simulink model "ground_sim"  (R2022a)
settings: Solver=FixedStepAuto  StartTime=0.0  StopTime=35  FixedStep=framePeriod_s  RelTol=1e-9
values from neighbouring files (symbols this model uses):
  framePeriod_s = 1/frameRate_hz    (= 0.02)    [autocode_setup.m]    (also in setup.m)
undefined symbols (not defined in the file or in its folder): accel_mps2, Aircraft, alt_msl_m, alt_wgs84_m, datetime, datevec, die_temp_c, Earth, Env, Fmu, gyro_radps, hdop, healthy, horz_acc_m, imu_healthy, InitCond, lat_rad, lon_rad, mag_healthy, mag_ut, ned_vel_mps, new_data, new_imu_data, new_mag_data, num_sats, pres_pa, spd_mps, Telem, tow_ms, track_acc_rad, track_rad, vdop, vel_acc_mps, vert_acc_m, week, WGS84
libraries: simulink x8, aerolibconvert2 x5, aerolibasang x3, aerolibtransform2 x2, aerolibgravity2 x2, aerolibatmos2 x1, sharedtransform x1, uavutilslib x1
(part 3 of 4)

== system ground_sim/Flight Management Unit/Vehicle Management System (VMS)/Variant Subsystem/FMU v1/Virtual to Non-Virtual Mapping1/Virtual to Non-Virtual Mapping2 ==
  Virtual : Inport
  Bus Creator : BusCreator  Inputs=new_imu_data,new_mag_data,imu_healthy,mag_healthy,die_temp_c,accel_mps2,gyro_radps,mag_ut  OutDataTypeStr=Bus: ImuData
  Bus Selector : BusSelector  OutputSignals=New IMU Data,New Magnetometer Data,IMU Healthy,Magnetometer Healthy,Die Temperature [C],Accelerometer [m/s/s],Gyro [rad/s],Magnetometer [uT]
  Data Type Conversion{,1..3} (4 alike) : DataTypeConversion  OutDataTypeStr=boolean  SaturateOnIntegerOverflow=off  RndMeth=Floor
  Data Type Conversion{4..7} (4 alike) : DataTypeConversion  OutDataTypeStr=single  SaturateOnIntegerOverflow=off  RndMeth=Floor
  Non-Virtual : Outport  OutDataTypeStr=Bus: ImuData
  wires:
  Bus Creator/1 -> Non-Virtual/1
  Virtual/1 -> Bus Selector/1
  Bus Selector/1 -> Data Type Conversion/1  "<New IMU Data>"
  Data Type Conversion/1 -> Bus Creator/1  "new_imu_data"
  Bus Selector/2 -> Data Type Conversion1/1  "<New Magnetometer Data>"
  Data Type Conversion1/1 -> Bus Creator/2  "new_mag_data"
  Bus Selector/3 -> Data Type Conversion2/1  "<IMU Healthy>"
  Data Type Conversion2/1 -> Bus Creator/3  "imu_healthy"
  Bus Selector/4 -> Data Type Conversion3/1  "<Magnetometer Healthy>"
  Data Type Conversion3/1 -> Bus Creator/4  "mag_healthy"
  Bus Selector/5 -> Data Type Conversion4/1  "<Die Temperature [C]>"
  Data Type Conversion4/1 -> Bus Creator/5  "die_temp_c"
  Bus Selector/6 -> Data Type Conversion5/1  "<Accelerometer [m/s/s]>"
  Bus Selector/7 -> Data Type Conversion6/1  "<Gyro [rad/s]>"
  Bus Selector/8 -> Data Type Conversion7/1  "<Magnetometer [uT]>"
  Data Type Conversion5/1 -> Bus Creator/6  "accel_mps2"
  Data Type Conversion6/1 -> Bus Creator/7  "gyro_radps"
  Data Type Conversion7/1 -> Bus Creator/8  "mag_ut"

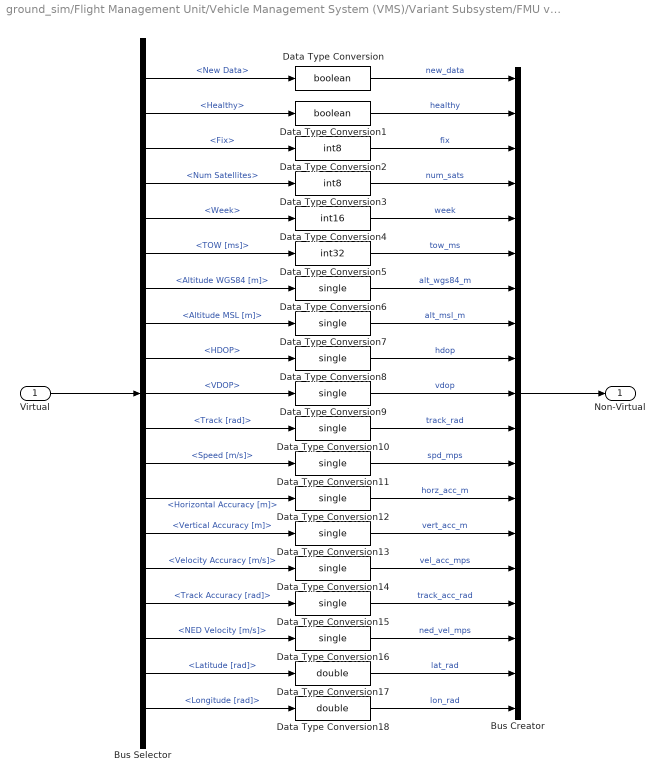
== system ground_sim/Flight Management Unit/Vehicle Management System (VMS)/Variant Subsystem/FMU v1/Virtual to Non-Virtual Mapping1/Virtual to Non-Virtual Mapping3 ==
  Virtual : Inport
  Bus Creator : BusCreator  Inputs=new_data,healthy,fix,num_sats,week,tow_ms,alt_wgs84_m,alt_msl_m,hdop,vdop,track_rad,spd_mps,horz_acc_m,vert_acc_m,vel_acc_mps,track_acc_rad,ned_vel_mps,lat_rad,lon_rad  OutDataTypeStr=Bus: GnssData
  Bus Selector : BusSelector  OutputSignals=New Data,Healthy,Fix,Num Satellites,Week,TOW [ms],Altitude WGS84 [m],Altitude MSL [m],HDOP,VDOP,Track [rad],Speed [m/s],Horizontal Accuracy [m],Vertical Accuracy [m],Velocity Accuracy [m/s],Track Accuracy [rad],NED Velocity [m/s],Latitude [rad],Longitude [rad]
  Data Type Conversion : DataTypeConversion  OutDataTypeStr=boolean  SaturateOnIntegerOverflow=off  RndMeth=Floor
  Data Type Conversion1 : DataTypeConversion  OutDataTypeStr=boolean  SaturateOnIntegerOverflow=off  RndMeth=Floor
  Data Type Conversion{6..16} (11 alike) : DataTypeConversion  OutDataTypeStr=single  SaturateOnIntegerOverflow=off  RndMeth=Floor
  Data Type Conversion17 : DataTypeConversion  OutDataTypeStr=double  SaturateOnIntegerOverflow=off  RndMeth=Floor
  Data Type Conversion18 : DataTypeConversion  OutDataTypeStr=double  SaturateOnIntegerOverflow=off  RndMeth=Floor
  Data Type Conversion2 : DataTypeConversion  OutDataTypeStr=int8  SaturateOnIntegerOverflow=off  RndMeth=Floor
  Data Type Conversion3 : DataTypeConversion  OutDataTypeStr=int8  SaturateOnIntegerOverflow=off  RndMeth=Floor
  Data Type Conversion4 : DataTypeConversion  OutDataTypeStr=int16  SaturateOnIntegerOverflow=off  RndMeth=Floor
  Data Type Conversion5 : DataTypeConversion  OutDataTypeStr=int32  SaturateOnIntegerOverflow=off  RndMeth=Floor
  Non-Virtual : Outport  OutDataTypeStr=Bus: GnssData
  wires:
  Virtual/1 -> Bus Selector/1
  Bus Creator/1 -> Non-Virtual/1
  Bus Selector/1 -> Data Type Conversion/1  "<New Data>"
  Data Type Conversion/1 -> Bus Creator/1  "new_data"
  Bus Selector/2 -> Data Type Conversion1/1  "<Healthy>"
  Data Type Conversion1/1 -> Bus Creator/2  "healthy"
  Bus Selector/3 -> Data Type Conversion2/1  "<Fix>"
  Data Type Conversion2/1 -> Bus Creator/3  "fix"
  Bus Selector/4 -> Data Type Conversion3/1  "<Num Satellites>"
  Data Type Conversion3/1 -> Bus Creator/4  "num_sats"
  Bus Selector/5 -> Data Type Conversion4/1  "<Week>"
  Data Type Conversion4/1 -> Bus Creator/5  "week"
  Bus Selector/6 -> Data Type Conversion5/1  "<TOW [ms]>"
  Data Type Conversion5/1 -> Bus Creator/6  "tow_ms"
  Bus Selector/7 -> Data Type Conversion6/1  "<Altitude WGS84 [m]>"
  Bus Selector/8 -> Data Type Conversion7/1  "<Altitude MSL [m]>"
  Data Type Conversion6/1 -> Bus Creator/7  "alt_wgs84_m"
  Data Type Conversion7/1 -> Bus Creator/8  "alt_msl_m"
  Bus Selector/9 -> Data Type Conversion8/1  "<HDOP>"
  Bus Selector/10 -> Data Type Conversion9/1  "<VDOP>"
  Data Type Conversion8/1 -> Bus Creator/9  "hdop"
  Data Type Conversion9/1 -> Bus Creator/10  "vdop"
  Bus Selector/11 -> Data Type Conversion10/1  "<Track [rad]>"
  Bus Selector/12 -> Data Type Conversion11/1  "<Speed [m/s]>"
  Data Type Conversion10/1 -> Bus Creator/11  "track_rad"
  Data Type Conversion11/1 -> Bus Creator/12  "spd_mps"
  Bus Selector/13 -> Data Type Conversion12/1  "<Horizontal Accuracy [m]>"
  Bus Selector/14 -> Data Type Conversion13/1  "<Vertical Accuracy [m]>"
  Bus Selector/15 -> Data Type Conversion14/1  "<Velocity Accuracy [m/s]>"
  Bus Selector/16 -> Data Type Conversion15/1  "<Track Accuracy [rad]>"
  Bus Selector/17 -> Data Type Conversion16/1  "<NED Velocity [m/s]>"
  Bus Selector/18 -> Data Type Conversion17/1  "<Latitude [rad]>"
  Bus Selector/19 -> Data Type Conversion18/1  "<Longitude [rad]>"
  Data Type Conversion18/1 -> Bus Creator/19  "lon_rad"
  Data Type Conversion17/1 -> Bus Creator/18  "lat_rad"
  Data Type Conversion16/1 -> Bus Creator/17  "ned_vel_mps"
  Data Type Conversion15/1 -> Bus Creator/16  "track_acc_rad"
  Data Type Conversion14/1 -> Bus Creator/15  "vel_acc_mps"
  Data Type Conversion13/1 -> Bus Creator/14  "vert_acc_m"
  Data Type Conversion12/1 -> Bus Creator/13  "horz_acc_m"

== system ground_sim/Flight Management Unit/Vehicle Management System (VMS)/Variant Subsystem/FMU v1/Virtual to Non-Virtual Mapping1/Virtual to Non-Virtual Mapping4 ==
  Virtual : Inport
  Bus Creator : BusCreator  Inputs=new_data,healthy,pres_pa,die_temp_c  OutDataTypeStr=Bus: PresData
  Bus Selector : BusSelector  OutputSignals=New Data,Healthy,Pressure [Pa],Die Temperature [C]
  Data Type Conversion : DataTypeConversion  OutDataTypeStr=boolean  SaturateOnIntegerOverflow=off  RndMeth=Floor
  Data Type Conversion1 : DataTypeConversion  OutDataTypeStr=boolean  SaturateOnIntegerOverflow=off  RndMeth=Floor
  Data Type Conversion2 : DataTypeConversion  OutDataTypeStr=single  SaturateOnIntegerOverflow=off  RndMeth=Floor
  Data Type Conversion3 : DataTypeConversion  OutDataTypeStr=single  SaturateOnIntegerOverflow=off  RndMeth=Floor
  Non-Virtual : Outport  OutDataTypeStr=Bus: PresData
  wires:
  Bus Creator/1 -> Non-Virtual/1
  Virtual/1 -> Bus Selector/1
  Bus Selector/1 -> Data Type Conversion/1  "<New Data>"
  Data Type Conversion/1 -> Bus Creator/1  "new_data"
  Bus Selector/2 -> Data Type Conversion1/1  "<Healthy>"
  Data Type Conversion1/1 -> Bus Creator/2  "healthy"
  Bus Selector/3 -> Data Type Conversion2/1  "<Pressure [Pa]>"
  Data Type Conversion2/1 -> Bus Creator/3  "pres_pa"
  Bus Selector/4 -> Data Type Conversion3/1  "<Die Temperature [C]>"
  Data Type Conversion3/1 -> Bus Creator/4  "die_temp_c"

== system ground_sim/Flight Management Unit/Vehicle Management System (VMS)/Variant Subsystem/FMU v1/Virtual to Non-Virtual Mapping1/Virtual to Non-Virtual Mapping5 ==
  Virtual : Inport
  Bus Creator : BusCreator  Inputs=new_data,healthy,pres_pa,die_temp_c  OutDataTypeStr=Bus: PresData
  Bus Selector : BusSelector  OutputSignals=New Data,Healthy,Pressure [Pa],Die Temperature [C]
  Data Type Conversion : DataTypeConversion  OutDataTypeStr=boolean  SaturateOnIntegerOverflow=off  RndMeth=Floor
  Data Type Conversion1 : DataTypeConversion  OutDataTypeStr=boolean  SaturateOnIntegerOverflow=off  RndMeth=Floor
  Data Type Conversion2 : DataTypeConversion  OutDataTypeStr=single  SaturateOnIntegerOverflow=off  RndMeth=Floor
  Data Type Conversion3 : DataTypeConversion  OutDataTypeStr=single  SaturateOnIntegerOverflow=off  RndMeth=Floor
  Non-Virtual : Outport  OutDataTypeStr=Bus: PresData
  wires:
  Data Type Conversion3/1 -> Bus Creator/4  "die_temp_c"
  Bus Selector/4 -> Data Type Conversion3/1  "<Die Temperature [C]>"
  Data Type Conversion2/1 -> Bus Creator/3  "pres_pa"
  Bus Selector/3 -> Data Type Conversion2/1  "<Pressure [Pa]>"
  Data Type Conversion1/1 -> Bus Creator/2  "healthy"
  Bus Selector/2 -> Data Type Conversion1/1  "<Healthy>"
  Data Type Conversion/1 -> Bus Creator/1  "new_data"
  Bus Selector/1 -> Data Type Conversion/1  "<New Data>"
  Virtual/1 -> Bus Selector/1
  Bus Creator/1 -> Non-Virtual/1

== system ground_sim/Flight Management Unit/Vehicle Management System (VMS)/Variant Subsystem/FMU v1/Virtual to Non-Virtual Mapping1/Virtual to Non-Virtual Mapping6 ==
  Virtual : Inport
  Bus Creator : BusCreator  Inputs=volt  OutDataTypeStr=Bus: AdcData
  Bus Selector : BusSelector  OutputSignals=Voltages
  Data Type Conversion2 : DataTypeConversion  OutDataTypeStr=single  SaturateOnIntegerOverflow=off  RndMeth=Floor
  Non-Virtual : Outport  OutDataTypeStr=Bus: AdcData
  wires:
  Bus Creator/1 -> Non-Virtual/1
  Virtual/1 -> Bus Selector/1
  Data Type Conversion2/1 -> Bus Creator/1  "volt"
  Bus Selector/1 -> Data Type Conversion2/1  "<Voltages>"

== system ground_sim/Flight Management Unit/Vehicle Management System (VMS)/Variant Subsystem/FMU v1/Virtual to Non-Virtual Mapping5/Subsystem2 ==
  Non-Virtual : Inport  OutDataTypeStr=Bus: AnalogData
  Bus Creator : BusCreator  Inputs=1
  Bus Selector : BusSelector  OutputSignals=val
  Data Type Conversion : DataTypeConversion  OutDataTypeStr=double  SaturateOnIntegerOverflow=off  RndMeth=Floor
  Virtual : Outport
  wires:
  Non-Virtual/1 -> Bus Selector/1
  Bus Creator/1 -> Virtual/1
  Data Type Conversion/1 -> Bus Creator/1  "Values"
  Bus Selector/1 -> Data Type Conversion/1  "<val>"

== system ground_sim/Flight Management Unit/Vehicle Management System (VMS)/Variant Subsystem/FMU v1/Virtual to Non-Virtual Mapping5/Subsystem3 ==
  Non-Virtual : Inport  OutDataTypeStr=Bus: PwmCmd
  Bus Creator : BusCreator  Inputs=2
  Bus Selector : BusSelector  OutputSignals=cnt,cmd
  Data Type Conversion : DataTypeConversion  OutDataTypeStr=double  SaturateOnIntegerOverflow=off  RndMeth=Floor
  Data Type Conversion1 : DataTypeConversion  OutDataTypeStr=double  SaturateOnIntegerOverflow=off  RndMeth=Floor
  Virtual : Outport
  wires:
  Non-Virtual/1 -> Bus Selector/1
  Bus Selector/2 -> Data Type Conversion1/1  "<cmd>"
  Data Type Conversion1/1 -> Bus Creator/2  "Cmds"
  Data Type Conversion/1 -> Bus Creator/1  "Counts"
  Bus Selector/1 -> Data Type Conversion/1  "<cnt>"
  Bus Creator/1 -> Virtual/1

== system ground_sim/Flight Management Unit/Vehicle Management System (VMS)/Variant Subsystem/FMU v1/Virtual to Non-Virtual Mapping5/Subsystem4 ==
  Non-Virtual : Inport  OutDataTypeStr=Bus: SbusCmd
  Bus Creator : BusCreator  Inputs=4
  Bus Selector : BusSelector  OutputSignals=ch17,ch18,cnt,cmd
  Data Type Conversion{,1..3} (4 alike) : DataTypeConversion  OutDataTypeStr=double  SaturateOnIntegerOverflow=off  RndMeth=Floor
  Virtual : Outport
  wires:
  Non-Virtual/1 -> Bus Selector/1
  Bus Creator/1 -> Virtual/1
  Bus Selector/1 -> Data Type Conversion/1  "<ch17>"
  Bus Selector/2 -> Data Type Conversion1/1  "<ch18>"
  Bus Selector/3 -> Data Type Conversion2/1  "<cnt>"
  Bus Selector/4 -> Data Type Conversion3/1  "<cmd>"
  Data Type Conversion2/1 -> Bus Creator/3  "Counts"
  Data Type Conversion3/1 -> Bus Creator/4  "Cmds"
  Data Type Conversion1/1 -> Bus Creator/2  "Ch 18"
  Data Type Conversion/1 -> Bus Creator/1  "Ch 17"

== system ground_sim/Flight Management Unit/Vehicle Management System (VMS)/Variant Subsystem/FMU v1/Virtual to Non-Virtual Mapping6/Virtual to Non-Virtual Mapping1 ==
  Virtual : Inport
  Bus Creator : BusCreator  Inputs=6
  Bus Selector : BusSelector  OutputSignals=New Data,Lost Frame,Failsafe,Ch 17,Ch 18,Channel Data
  Data Type Conversion{,1..4} (5 alike) : DataTypeConversion  OutDataTypeStr=boolean  SaturateOnIntegerOverflow=off  RndMeth=Floor
  Data Type Conversion5 : DataTypeConversion  OutDataTypeStr=int16  SaturateOnIntegerOverflow=off  RndMeth=Floor
  Non-Virtual : Outport  OutDataTypeStr=Bus: InceptorData
  wires:
  Virtual/1 -> Bus Selector/1
  Bus Creator/1 -> Non-Virtual/1
  Bus Selector/1 -> Data Type Conversion/1  "<New Data>"
  Bus Selector/2 -> Data Type Conversion1/1  "<Lost Frame>"
  Bus Selector/3 -> Data Type Conversion2/1  "<Failsafe>"
  Bus Selector/4 -> Data Type Conversion3/1  "<Ch 17>"
  Bus Selector/5 -> Data Type Conversion4/1  "<Ch 18>"
  Bus Selector/6 -> Data Type Conversion5/1  "<Channel Data>"
  Data Type Conversion/1 -> Bus Creator/1  "new_data"
  Data Type Conversion1/1 -> Bus Creator/2  "lost_frame"
  Data Type Conversion2/1 -> Bus Creator/3  "failsafe"
  Data Type Conversion3/1 -> Bus Creator/4  "ch17"
  Data Type Conversion4/1 -> Bus Creator/5  "ch18"
  Data Type Conversion5/1 -> Bus Creator/6  "ch"

== system ground_sim/Flight Management Unit/Vehicle Management System (VMS)/Variant Subsystem/FMU v1/Virtual to Non-Virtual Mapping6/Virtual to Non-Virtual Mapping2 ==
  Virtual : Inport
  Bus Creator : BusCreator  Inputs=8
  Bus Selector : BusSelector  OutputSignals=New IMU Data,New Magnetometer Data,IMU Healthy,Magnetometer Healthy,Die Temperature [C],Accelerometer [m/s/s],Gyro [rad/s],Magnetometer [uT]
  Data Type Conversion{,1..3} (4 alike) : DataTypeConversion  OutDataTypeStr=boolean  SaturateOnIntegerOverflow=off  RndMeth=Floor
  Data Type Conversion{4..7} (4 alike) : DataTypeConversion  OutDataTypeStr=single  SaturateOnIntegerOverflow=off  RndMeth=Floor
  Non-Virtual : Outport  OutDataTypeStr=Bus: ImuData
  wires:
  Bus Creator/1 -> Non-Virtual/1
  Virtual/1 -> Bus Selector/1
  Bus Selector/1 -> Data Type Conversion/1  "<New IMU Data>"
  Data Type Conversion/1 -> Bus Creator/1  "new_imu_data"
  Bus Selector/2 -> Data Type Conversion1/1  "<New Magnetometer Data>"
  Data Type Conversion1/1 -> Bus Creator/2  "new_mag_data"
  Bus Selector/3 -> Data Type Conversion2/1  "<IMU Healthy>"
  Data Type Conversion2/1 -> Bus Creator/3  "imu_healthy"
  Bus Selector/4 -> Data Type Conversion3/1  "<Magnetometer Healthy>"
  Data Type Conversion3/1 -> Bus Creator/4  "mag_healthy"
  Bus Selector/5 -> Data Type Conversion4/1  "<Die Temperature [C]>"
  Data Type Conversion4/1 -> Bus Creator/5  "die_temp_c"
  Bus Selector/6 -> Data Type Conversion5/1  "<Accelerometer [m/s/s]>"
  Bus Selector/7 -> Data Type Conversion6/1  "<Gyro [rad/s]>"
  Bus Selector/8 -> Data Type Conversion7/1  "<Magnetometer [uT]>"
  Data Type Conversion5/1 -> Bus Creator/6  "accel_mps2"
  Data Type Conversion6/1 -> Bus Creator/7  "gyro_radps"
  Data Type Conversion7/1 -> Bus Creator/8  "mag_ut"

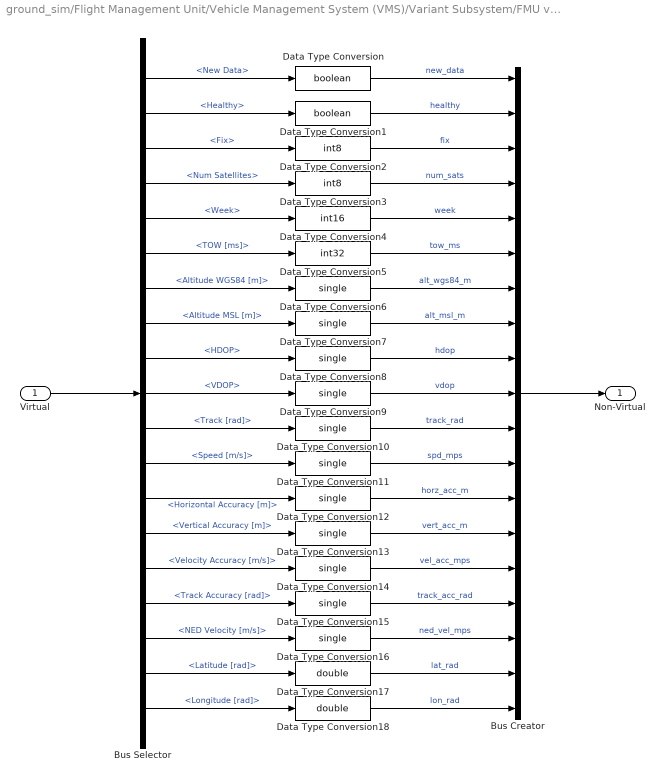
== system ground_sim/Flight Management Unit/Vehicle Management System (VMS)/Variant Subsystem/FMU v1/Virtual to Non-Virtual Mapping6/Virtual to Non-Virtual Mapping3 ==
  Virtual : Inport
  Bus Creator : BusCreator  Inputs=19
  Bus Selector : BusSelector  OutputSignals=New Data,Healthy,Fix,Num Satellites,Week,TOW [ms],Altitude WGS84 [m],Altitude MSL [m],HDOP,VDOP,Track [rad],Speed [m/s],Horizontal Accuracy [m],Vertical Accuracy [m],Velocity Accuracy [m/s],Track Accuracy [rad],NED Velocity [m/s],Latitude [rad],Longitude [rad]
  Data Type Conversion : DataTypeConversion  OutDataTypeStr=boolean  SaturateOnIntegerOverflow=off  RndMeth=Floor
  Data Type Conversion1 : DataTypeConversion  OutDataTypeStr=boolean  SaturateOnIntegerOverflow=off  RndMeth=Floor
  Data Type Conversion{6..16} (11 alike) : DataTypeConversion  OutDataTypeStr=single  SaturateOnIntegerOverflow=off  RndMeth=Floor
  Data Type Conversion17 : DataTypeConversion  OutDataTypeStr=double  SaturateOnIntegerOverflow=off  RndMeth=Floor
  Data Type Conversion18 : DataTypeConversion  OutDataTypeStr=double  SaturateOnIntegerOverflow=off  RndMeth=Floor
  Data Type Conversion2 : DataTypeConversion  OutDataTypeStr=int8  SaturateOnIntegerOverflow=off  RndMeth=Floor
  Data Type Conversion3 : DataTypeConversion  OutDataTypeStr=int8  SaturateOnIntegerOverflow=off  RndMeth=Floor
  Data Type Conversion4 : DataTypeConversion  OutDataTypeStr=int16  SaturateOnIntegerOverflow=off  RndMeth=Floor
  Data Type Conversion5 : DataTypeConversion  OutDataTypeStr=int32  SaturateOnIntegerOverflow=off  RndMeth=Floor
  Non-Virtual : Outport  OutDataTypeStr=Bus: GnssData
  wires:
  Virtual/1 -> Bus Selector/1
  Bus Creator/1 -> Non-Virtual/1
  Bus Selector/1 -> Data Type Conversion/1  "<New Data>"
  Data Type Conversion/1 -> Bus Creator/1  "new_data"
  Bus Selector/2 -> Data Type Conversion1/1  "<Healthy>"
  Data Type Conversion1/1 -> Bus Creator/2  "healthy"
  Bus Selector/3 -> Data Type Conversion2/1  "<Fix>"
  Data Type Conversion2/1 -> Bus Creator/3  "fix"
  Bus Selector/4 -> Data Type Conversion3/1  "<Num Satellites>"
  Data Type Conversion3/1 -> Bus Creator/4  "num_sats"
  Bus Selector/5 -> Data Type Conversion4/1  "<Week>"
  Data Type Conversion4/1 -> Bus Creator/5  "week"
  Bus Selector/6 -> Data Type Conversion5/1  "<TOW [ms]>"
  Data Type Conversion5/1 -> Bus Creator/6  "tow_ms"
  Bus Selector/7 -> Data Type Conversion6/1  "<Altitude WGS84 [m]>"
  Bus Selector/8 -> Data Type Conversion7/1  "<Altitude MSL [m]>"
  Data Type Conversion6/1 -> Bus Creator/7  "alt_wgs84_m"
  Data Type Conversion7/1 -> Bus Creator/8  "alt_msl_m"
  Bus Selector/9 -> Data Type Conversion8/1  "<HDOP>"
  Bus Selector/10 -> Data Type Conversion9/1  "<VDOP>"
  Data Type Conversion8/1 -> Bus Creator/9  "hdop"
  Data Type Conversion9/1 -> Bus Creator/10  "vdop"
  Bus Selector/11 -> Data Type Conversion10/1  "<Track [rad]>"
  Bus Selector/12 -> Data Type Conversion11/1  "<Speed [m/s]>"
  Data Type Conversion10/1 -> Bus Creator/11  "track_rad"
  Data Type Conversion11/1 -> Bus Creator/12  "spd_mps"
  Bus Selector/13 -> Data Type Conversion12/1  "<Horizontal Accuracy [m]>"
  Bus Selector/14 -> Data Type Conversion13/1  "<Vertical Accuracy [m]>"
  Bus Selector/15 -> Data Type Conversion14/1  "<Velocity Accuracy [m/s]>"
  Bus Selector/16 -> Data Type Conversion15/1  "<Track Accuracy [rad]>"
  Bus Selector/17 -> Data Type Conversion16/1  "<NED Velocity [m/s]>"
  Bus Selector/18 -> Data Type Conversion17/1  "<Latitude [rad]>"
  Bus Selector/19 -> Data Type Conversion18/1  "<Longitude [rad]>"
  Data Type Conversion18/1 -> Bus Creator/19  "lon_rad"
  Data Type Conversion17/1 -> Bus Creator/18  "lat_rad"
  Data Type Conversion16/1 -> Bus Creator/17  "ned_vel_mps"
  Data Type Conversion15/1 -> Bus Creator/16  "track_acc_rad"
  Data Type Conversion14/1 -> Bus Creator/15  "vel_acc_mps"
  Data Type Conversion13/1 -> Bus Creator/14  "vert_acc_m"
  Data Type Conversion12/1 -> Bus Creator/13  "horz_acc_m"

== system ground_sim/Flight Management Unit/Vehicle Management System (VMS)/Variant Subsystem/FMU v1/Virtual to Non-Virtual Mapping6/Virtual to Non-Virtual Mapping4 ==
  Virtual : Inport
  Bus Creator : BusCreator  Inputs=4
  Bus Selector : BusSelector  OutputSignals=New Data,Healthy,Pressure [Pa],Die Temperature [C]
  Data Type Conversion : DataTypeConversion  OutDataTypeStr=boolean  SaturateOnIntegerOverflow=off  RndMeth=Floor
  Data Type Conversion1 : DataTypeConversion  OutDataTypeStr=boolean  SaturateOnIntegerOverflow=off  RndMeth=Floor
  Data Type Conversion2 : DataTypeConversion  OutDataTypeStr=single  SaturateOnIntegerOverflow=off  RndMeth=Floor
  Data Type Conversion3 : DataTypeConversion  OutDataTypeStr=single  SaturateOnIntegerOverflow=off  RndMeth=Floor
  Non-Virtual : Outport  OutDataTypeStr=Bus: PresData
  wires:
  Bus Creator/1 -> Non-Virtual/1
  Virtual/1 -> Bus Selector/1
  Bus Selector/1 -> Data Type Conversion/1  "<New Data>"
  Data Type Conversion/1 -> Bus Creator/1  "new_data"
  Bus Selector/2 -> Data Type Conversion1/1  "<Healthy>"
  Data Type Conversion1/1 -> Bus Creator/2  "healthy"
  Bus Selector/3 -> Data Type Conversion2/1  "<Pressure [Pa]>"
  Data Type Conversion2/1 -> Bus Creator/3  "pres_pa"
  Bus Selector/4 -> Data Type Conversion3/1  "<Die Temperature [C]>"
  Data Type Conversion3/1 -> Bus Creator/4  "die_temp_c"

== system ground_sim/Flight Management Unit/Vehicle Management System (VMS)/Variant Subsystem/FMU v1/Virtual to Non-Virtual Mapping6/Virtual to Non-Virtual Mapping5 ==
  Virtual : Inport
  Bus Creator : BusCreator  Inputs=4
  Bus Selector : BusSelector  OutputSignals=New Data,Healthy,Pressure [Pa],Die Temperature [C]
  Data Type Conversion : DataTypeConversion  OutDataTypeStr=boolean  SaturateOnIntegerOverflow=off  RndMeth=Floor
  Data Type Conversion1 : DataTypeConversion  OutDataTypeStr=boolean  SaturateOnIntegerOverflow=off  RndMeth=Floor
  Data Type Conversion2 : DataTypeConversion  OutDataTypeStr=single  SaturateOnIntegerOverflow=off  RndMeth=Floor
  Data Type Conversion3 : DataTypeConversion  OutDataTypeStr=single  SaturateOnIntegerOverflow=off  RndMeth=Floor
  Non-Virtual : Outport  OutDataTypeStr=Bus: PresData
  wires:
  Data Type Conversion3/1 -> Bus Creator/4  "die_temp_c"
  Bus Selector/4 -> Data Type Conversion3/1  "<Die Temperature [C]>"
  Data Type Conversion2/1 -> Bus Creator/3  "pres_pa"
  Bus Selector/3 -> Data Type Conversion2/1  "<Pressure [Pa]>"
  Data Type Conversion1/1 -> Bus Creator/2  "healthy"
  Bus Selector/2 -> Data Type Conversion1/1  "<Healthy>"
  Data Type Conversion/1 -> Bus Creator/1  "new_data"
  Bus Selector/1 -> Data Type Conversion/1  "<New Data>"
  Virtual/1 -> Bus Selector/1
  Bus Creator/1 -> Non-Virtual/1

== system ground_sim/Flight Management Unit/Vehicle Management System (VMS)/Variant Subsystem/FMU v1/Virtual to Non-Virtual Mapping6/Virtual to Non-Virtual Mapping6 ==
  Virtual : Inport
  Bus Creator : BusCreator  Inputs=1
  Bus Selector : BusSelector  OutputSignals=Voltages
  Data Type Conversion2 : DataTypeConversion  OutDataTypeStr=single  SaturateOnIntegerOverflow=off  RndMeth=Floor
  Non-Virtual : Outport  OutDataTypeStr=Bus: AdcData
  wires:
  Bus Creator/1 -> Non-Virtual/1
  Virtual/1 -> Bus Selector/1
  Data Type Conversion2/1 -> Bus Creator/1  "volt"
  Bus Selector/1 -> Data Type Conversion2/1  "<Voltages>"

== system ground_sim/Flight Management Unit/Vehicle Management System (VMS)/Variant Subsystem/FMU v1/Virtual to Non-Virtual Mapping6/Virtual to Non-Virtual Mapping7 ==
  Virtual : Inport
  Bus Creator : BusCreator  Inputs=2
  Bus Selector : BusSelector  OutputSignals=Voltage [V],Current [V]
  Data Type Conversion1 : DataTypeConversion  OutDataTypeStr=single  SaturateOnIntegerOverflow=off  RndMeth=Floor
  Data Type Conversion2 : DataTypeConversion  OutDataTypeStr=single  SaturateOnIntegerOverflow=off  RndMeth=Floor
  Non-Virtual : Outport  OutDataTypeStr=Bus: PowerModuleData
  wires:
  Virtual/1 -> Bus Selector/1
  Bus Creator/1 -> Non-Virtual/1
  Bus Selector/1 -> Data Type Conversion1/1  "<Voltage [V]>"
  Data Type Conversion1/1 -> Bus Creator/1  "voltage_v"
  Bus Selector/2 -> Data Type Conversion2/1  "<Current [V]>"
  Data Type Conversion2/1 -> Bus Creator/2  "current_v"

== system ground_sim/Flight Management Unit/Vehicle Management System (VMS)/Variant Subsystem/FMU v2/Virtual to Non-Virtual Mapping1/Virtual to Non-Virtual Mapping1 ==
  Virtual : Inport
  Bus Creator : BusCreator  Inputs=6
  Bus Selector : BusSelector  OutputSignals=New Data,Lost Frame,Failsafe,Ch 17,Ch 18,Channel Data
  Data Type Conversion{,1..4} (5 alike) : DataTypeConversion  OutDataTypeStr=boolean  SaturateOnIntegerOverflow=off  RndMeth=Floor
  Data Type Conversion5 : DataTypeConversion  OutDataTypeStr=int16  SaturateOnIntegerOverflow=off  RndMeth=Floor
  Non-Virtual : Outport  OutDataTypeStr=Bus: InceptorData
  wires:
  Virtual/1 -> Bus Selector/1
  Bus Creator/1 -> Non-Virtual/1
  Bus Selector/1 -> Data Type Conversion/1  "<New Data>"
  Bus Selector/2 -> Data Type Conversion1/1  "<Lost Frame>"
  Bus Selector/3 -> Data Type Conversion2/1  "<Failsafe>"
  Bus Selector/4 -> Data Type Conversion3/1  "<Ch 17>"
  Bus Selector/5 -> Data Type Conversion4/1  "<Ch 18>"
  Bus Selector/6 -> Data Type Conversion5/1  "<Channel Data>"
  Data Type Conversion/1 -> Bus Creator/1  "new_data"
  Data Type Conversion1/1 -> Bus Creator/2  "lost_frame"
  Data Type Conversion2/1 -> Bus Creator/3  "failsafe"
  Data Type Conversion3/1 -> Bus Creator/4  "ch17"
  Data Type Conversion4/1 -> Bus Creator/5  "ch18"
  Data Type Conversion5/1 -> Bus Creator/6  "ch"

== system ground_sim/Flight Management Unit/Vehicle Management System (VMS)/Variant Subsystem/FMU v2/Virtual to Non-Virtual Mapping1/Virtual to Non-Virtual Mapping2 ==
  Virtual : Inport
  Bus Creator : BusCreator  Inputs=8
  Bus Selector : BusSelector  OutputSignals=New IMU Data,New Magnetometer Data,IMU Healthy,Magnetometer Healthy,Die Temperature [C],Accelerometer [m/s/s],Gyro [rad/s],Magnetometer [uT]
  Data Type Conversion{,1..3} (4 alike) : DataTypeConversion  OutDataTypeStr=boolean  SaturateOnIntegerOverflow=off  RndMeth=Floor
  Data Type Conversion{4..7} (4 alike) : DataTypeConversion  OutDataTypeStr=single  SaturateOnIntegerOverflow=off  RndMeth=Floor
  Non-Virtual : Outport  OutDataTypeStr=Bus: ImuData
  wires:
  Bus Creator/1 -> Non-Virtual/1
  Virtual/1 -> Bus Selector/1
  Bus Selector/1 -> Data Type Conversion/1  "<New IMU Data>"
  Data Type Conversion/1 -> Bus Creator/1  "new_imu_data"
  Bus Selector/2 -> Data Type Conversion1/1  "<New Magnetometer Data>"
  Data Type Conversion1/1 -> Bus Creator/2  "new_mag_data"
  Bus Selector/3 -> Data Type Conversion2/1  "<IMU Healthy>"
  Data Type Conversion2/1 -> Bus Creator/3  "imu_healthy"
  Bus Selector/4 -> Data Type Conversion3/1  "<Magnetometer Healthy>"
  Data Type Conversion3/1 -> Bus Creator/4  "mag_healthy"
  Bus Selector/5 -> Data Type Conversion4/1  "<Die Temperature [C]>"
  Data Type Conversion4/1 -> Bus Creator/5  "die_temp_c"
  Bus Selector/6 -> Data Type Conversion5/1  "<Accelerometer [m/s/s]>"
  Bus Selector/7 -> Data Type Conversion6/1  "<Gyro [rad/s]>"
  Bus Selector/8 -> Data Type Conversion7/1  "<Magnetometer [uT]>"
  Data Type Conversion5/1 -> Bus Creator/6  "accel_mps2"
  Data Type Conversion6/1 -> Bus Creator/7  "gyro_radps"
  Data Type Conversion7/1 -> Bus Creator/8  "mag_ut"

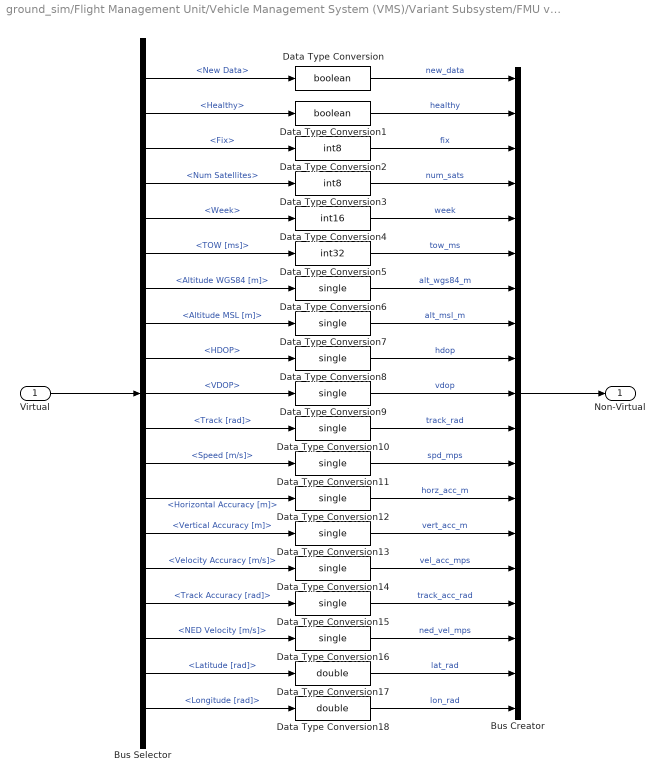
== system ground_sim/Flight Management Unit/Vehicle Management System (VMS)/Variant Subsystem/FMU v2/Virtual to Non-Virtual Mapping1/Virtual to Non-Virtual Mapping3 ==
  Virtual : Inport
  Bus Creator : BusCreator  Inputs=19
  Bus Selector : BusSelector  OutputSignals=New Data,Healthy,Fix,Num Satellites,Week,TOW [ms],Altitude WGS84 [m],Altitude MSL [m],HDOP,VDOP,Track [rad],Speed [m/s],Horizontal Accuracy [m],Vertical Accuracy [m],Velocity Accuracy [m/s],Track Accuracy [rad],NED Velocity [m/s],Latitude [rad],Longitude [rad]
  Data Type Conversion : DataTypeConversion  OutDataTypeStr=boolean  SaturateOnIntegerOverflow=off  RndMeth=Floor
  Data Type Conversion1 : DataTypeConversion  OutDataTypeStr=boolean  SaturateOnIntegerOverflow=off  RndMeth=Floor
  Data Type Conversion{6..16} (11 alike) : DataTypeConversion  OutDataTypeStr=single  SaturateOnIntegerOverflow=off  RndMeth=Floor
  Data Type Conversion17 : DataTypeConversion  OutDataTypeStr=double  SaturateOnIntegerOverflow=off  RndMeth=Floor
  Data Type Conversion18 : DataTypeConversion  OutDataTypeStr=double  SaturateOnIntegerOverflow=off  RndMeth=Floor
  Data Type Conversion2 : DataTypeConversion  OutDataTypeStr=int8  SaturateOnIntegerOverflow=off  RndMeth=Floor
  Data Type Conversion3 : DataTypeConversion  OutDataTypeStr=int8  SaturateOnIntegerOverflow=off  RndMeth=Floor
  Data Type Conversion4 : DataTypeConversion  OutDataTypeStr=int16  SaturateOnIntegerOverflow=off  RndMeth=Floor
  Data Type Conversion5 : DataTypeConversion  OutDataTypeStr=int32  SaturateOnIntegerOverflow=off  RndMeth=Floor
  Non-Virtual : Outport  OutDataTypeStr=Bus: GnssData
  wires:
  Virtual/1 -> Bus Selector/1
  Bus Creator/1 -> Non-Virtual/1
  Bus Selector/1 -> Data Type Conversion/1  "<New Data>"
  Data Type Conversion/1 -> Bus Creator/1  "new_data"
  Bus Selector/2 -> Data Type Conversion1/1  "<Healthy>"
  Data Type Conversion1/1 -> Bus Creator/2  "healthy"
  Bus Selector/3 -> Data Type Conversion2/1  "<Fix>"
  Data Type Conversion2/1 -> Bus Creator/3  "fix"
  Bus Selector/4 -> Data Type Conversion3/1  "<Num Satellites>"
  Data Type Conversion3/1 -> Bus Creator/4  "num_sats"
  Bus Selector/5 -> Data Type Conversion4/1  "<Week>"
  Data Type Conversion4/1 -> Bus Creator/5  "week"
  Bus Selector/6 -> Data Type Conversion5/1  "<TOW [ms]>"
  Data Type Conversion5/1 -> Bus Creator/6  "tow_ms"
  Bus Selector/7 -> Data Type Conversion6/1  "<Altitude WGS84 [m]>"
  Bus Selector/8 -> Data Type Conversion7/1  "<Altitude MSL [m]>"
  Data Type Conversion6/1 -> Bus Creator/7  "alt_wgs84_m"
  Data Type Conversion7/1 -> Bus Creator/8  "alt_msl_m"
  Bus Selector/9 -> Data Type Conversion8/1  "<HDOP>"
  Bus Selector/10 -> Data Type Conversion9/1  "<VDOP>"
  Data Type Conversion8/1 -> Bus Creator/9  "hdop"
  Data Type Conversion9/1 -> Bus Creator/10  "vdop"
  Bus Selector/11 -> Data Type Conversion10/1  "<Track [rad]>"
  Bus Selector/12 -> Data Type Conversion11/1  "<Speed [m/s]>"
  Data Type Conversion10/1 -> Bus Creator/11  "track_rad"
  Data Type Conversion11/1 -> Bus Creator/12  "spd_mps"
  Bus Selector/13 -> Data Type Conversion12/1  "<Horizontal Accuracy [m]>"
  Bus Selector/14 -> Data Type Conversion13/1  "<Vertical Accuracy [m]>"
  Bus Selector/15 -> Data Type Conversion14/1  "<Velocity Accuracy [m/s]>"
  Bus Selector/16 -> Data Type Conversion15/1  "<Track Accuracy [rad]>"
  Bus Selector/17 -> Data Type Conversion16/1  "<NED Velocity [m/s]>"
  Bus Selector/18 -> Data Type Conversion17/1  "<Latitude [rad]>"
  Bus Selector/19 -> Data Type Conversion18/1  "<Longitude [rad]>"
  Data Type Conversion18/1 -> Bus Creator/19  "lon_rad"
  Data Type Conversion17/1 -> Bus Creator/18  "lat_rad"
  Data Type Conversion16/1 -> Bus Creator/17  "ned_vel_mps"
  Data Type Conversion15/1 -> Bus Creator/16  "track_acc_rad"
  Data Type Conversion14/1 -> Bus Creator/15  "vel_acc_mps"
  Data Type Conversion13/1 -> Bus Creator/14  "vert_acc_m"
  Data Type Conversion12/1 -> Bus Creator/13  "horz_acc_m"

== system ground_sim/Flight Management Unit/Vehicle Management System (VMS)/Variant Subsystem/FMU v2/Virtual to Non-Virtual Mapping1/Virtual to Non-Virtual Mapping4 ==
  Virtual : Inport
  Bus Creator : BusCreator  Inputs=4
  Bus Selector : BusSelector  OutputSignals=New Data,Healthy,Pressure [Pa],Die Temperature [C]
  Data Type Conversion : DataTypeConversion  OutDataTypeStr=boolean  SaturateOnIntegerOverflow=off  RndMeth=Floor
  Data Type Conversion1 : DataTypeConversion  OutDataTypeStr=boolean  SaturateOnIntegerOverflow=off  RndMeth=Floor
  Data Type Conversion2 : DataTypeConversion  OutDataTypeStr=single  SaturateOnIntegerOverflow=off  RndMeth=Floor
  Data Type Conversion3 : DataTypeConversion  OutDataTypeStr=single  SaturateOnIntegerOverflow=off  RndMeth=Floor
  Non-Virtual : Outport  OutDataTypeStr=Bus: PresData
  wires:
  Bus Creator/1 -> Non-Virtual/1
  Virtual/1 -> Bus Selector/1
  Bus Selector/1 -> Data Type Conversion/1  "<New Data>"
  Data Type Conversion/1 -> Bus Creator/1  "new_data"
  Bus Selector/2 -> Data Type Conversion1/1  "<Healthy>"
  Data Type Conversion1/1 -> Bus Creator/2  "healthy"
  Bus Selector/3 -> Data Type Conversion2/1  "<Pressure [Pa]>"
  Data Type Conversion2/1 -> Bus Creator/3  "pres_pa"
  Bus Selector/4 -> Data Type Conversion3/1  "<Die Temperature [C]>"
  Data Type Conversion3/1 -> Bus Creator/4  "die_temp_c"

== system ground_sim/Flight Management Unit/Vehicle Management System (VMS)/Variant Subsystem/FMU v2/Virtual to Non-Virtual Mapping1/Virtual to Non-Virtual Mapping5 ==
  Virtual : Inport
  Bus Creator : BusCreator  Inputs=4
  Bus Selector : BusSelector  OutputSignals=New Data,Healthy,Pressure [Pa],Die Temperature [C]
  Data Type Conversion : DataTypeConversion  OutDataTypeStr=boolean  SaturateOnIntegerOverflow=off  RndMeth=Floor
  Data Type Conversion1 : DataTypeConversion  OutDataTypeStr=boolean  SaturateOnIntegerOverflow=off  RndMeth=Floor
  Data Type Conversion2 : DataTypeConversion  OutDataTypeStr=single  SaturateOnIntegerOverflow=off  RndMeth=Floor
  Data Type Conversion3 : DataTypeConversion  OutDataTypeStr=single  SaturateOnIntegerOverflow=off  RndMeth=Floor
  Non-Virtual : Outport  OutDataTypeStr=Bus: PresData
  wires:
  Data Type Conversion3/1 -> Bus Creator/4  "die_temp_c"
  Bus Selector/4 -> Data Type Conversion3/1  "<Die Temperature [C]>"
  Data Type Conversion2/1 -> Bus Creator/3  "pres_pa"
  Bus Selector/3 -> Data Type Conversion2/1  "<Pressure [Pa]>"
  Data Type Conversion1/1 -> Bus Creator/2  "healthy"
  Bus Selector/2 -> Data Type Conversion1/1  "<Healthy>"
  Data Type Conversion/1 -> Bus Creator/1  "new_data"
  Bus Selector/1 -> Data Type Conversion/1  "<New Data>"
  Virtual/1 -> Bus Selector/1
  Bus Creator/1 -> Non-Virtual/1

== system ground_sim/Flight Management Unit/Vehicle Management System (VMS)/Variant Subsystem/FMU v2/Virtual to Non-Virtual Mapping1/Virtual to Non-Virtual Mapping6 ==
  Virtual : Inport
  Bus Creator : BusCreator  Inputs=1
  Bus Selector : BusSelector  OutputSignals=Voltages
  Data Type Conversion2 : DataTypeConversion  OutDataTypeStr=single  SaturateOnIntegerOverflow=off  RndMeth=Floor
  Non-Virtual : Outport  OutDataTypeStr=Bus: AdcData
  wires:
  Bus Creator/1 -> Non-Virtual/1
  Virtual/1 -> Bus Selector/1
  Data Type Conversion2/1 -> Bus Creator/1  "volt"
  Bus Selector/1 -> Data Type Conversion2/1  "<Voltages>"

== system ground_sim/Flight Management Unit/Vehicle Management System (VMS)/Variant Subsystem/FMU v2/Virtual to Non-Virtual Mapping1/Virtual to Non-Virtual Mapping7 ==
  Virtual : Inport
  Bus Creator : BusCreator  Inputs=2
  Bus Selector : BusSelector  OutputSignals=Voltage [V],Current [V]
  Data Type Conversion1 : DataTypeConversion  OutDataTypeStr=single  SaturateOnIntegerOverflow=off  RndMeth=Floor
  Data Type Conversion2 : DataTypeConversion  OutDataTypeStr=single  SaturateOnIntegerOverflow=off  RndMeth=Floor
  Non-Virtual : Outport  OutDataTypeStr=Bus: PowerModuleData
  wires:
  Virtual/1 -> Bus Selector/1
  Bus Creator/1 -> Non-Virtual/1
  Bus Selector/1 -> Data Type Conversion1/1  "<Voltage [V]>"
  Data Type Conversion1/1 -> Bus Creator/1  "voltage_v"
  Bus Selector/2 -> Data Type Conversion2/1  "<Current [V]>"
  Data Type Conversion2/1 -> Bus Creator/2  "current_v"

== system ground_sim/Flight Management Unit/Vehicle Management System (VMS)/Variant Subsystem/FMU v2/Virtual to Non-Virtual Mapping4/Subsystem1 ==
  Non-Virtual : Inport  OutDataTypeStr=Bus: BatteryData
  Bus Creator : BusCreator  Inputs=5
  Bus Selector : BusSelector  OutputSignals=voltage_v,current_ma,consumed_mah,remaining_prcnt,remaining_time_s
  Data Type Conversion{,1..4} (5 alike) : DataTypeConversion  OutDataTypeStr=double  SaturateOnIntegerOverflow=off  RndMeth=Floor
  Virtual : Outport
  wires:
  Non-Virtual/1 -> Bus Selector/1
  Bus Selector/1 -> Data Type Conversion/1  "<voltage_v>"
  Bus Selector/2 -> Data Type Conversion1/1  "<current_ma>"
  Bus Selector/3 -> Data Type Conversion2/1  "<consumed_mah>"
  Bus Selector/4 -> Data Type Conversion3/1  "<remaining_prcnt>"
  Bus Selector/5 -> Data Type Conversion4/1  "<remaining_time_s>"
  Bus Creator/1 -> Virtual/1
  Data Type Conversion/1 -> Bus Creator/1  "Voltage [V]"
  Data Type Conversion1/1 -> Bus Creator/2  "Current [mA]"
  Data Type Conversion2/1 -> Bus Creator/3  "Consumed Capacity [mAh]"
  Data Type Conversion3/1 -> Bus Creator/4  "Remaining Capacity [%]"
  Data Type Conversion4/1 -> Bus Creator/5  "Remaining Flight Time [s]"

== system ground_sim/Flight Management Unit/Vehicle Management System (VMS)/Variant Subsystem/FMU v2/Virtual to Non-Virtual Mapping4/Subsystem2 ==
  Non-Virtual : Inport  OutDataTypeStr=Bus: AnalogData
  Bus Creator : BusCreator  Inputs=1
  Bus Selector : BusSelector  OutputSignals=val
  Data Type Conversion : DataTypeConversion  OutDataTypeStr=double  SaturateOnIntegerOverflow=off  RndMeth=Floor
  Virtual : Outport
  wires:
  Non-Virtual/1 -> Bus Selector/1
  Bus Creator/1 -> Virtual/1
  Data Type Conversion/1 -> Bus Creator/1  "Values"
  Bus Selector/1 -> Data Type Conversion/1  "<val>"

== system ground_sim/Flight Management Unit/Vehicle Management System (VMS)/Variant Subsystem/FMU v2/Virtual to Non-Virtual Mapping4/Subsystem3 ==
  Non-Virtual : Inport  OutDataTypeStr=Bus: PwmCmd
  Bus Creator : BusCreator  Inputs=2
  Bus Selector : BusSelector  OutputSignals=cnt,cmd
  Data Type Conversion : DataTypeConversion  OutDataTypeStr=double  SaturateOnIntegerOverflow=off  RndMeth=Floor
  Data Type Conversion1 : DataTypeConversion  OutDataTypeStr=double  SaturateOnIntegerOverflow=off  RndMeth=Floor
  Virtual : Outport
  wires:
  Non-Virtual/1 -> Bus Selector/1
  Bus Selector/2 -> Data Type Conversion1/1  "<cmd>"
  Data Type Conversion1/1 -> Bus Creator/2  "Cmds"
  Data Type Conversion/1 -> Bus Creator/1  "Counts"
  Bus Selector/1 -> Data Type Conversion/1  "<cnt>"
  Bus Creator/1 -> Virtual/1

== system ground_sim/Flight Management Unit/Vehicle Management System (VMS)/Variant Subsystem/FMU v2/Virtual to Non-Virtual Mapping4/Subsystem4 ==
  Non-Virtual : Inport  OutDataTypeStr=Bus: SbusCmd
  Bus Creator : BusCreator  Inputs=4
  Bus Selector : BusSelector  OutputSignals=ch17,ch18,cnt,cmd
  Data Type Conversion{,1..3} (4 alike) : DataTypeConversion  OutDataTypeStr=double  SaturateOnIntegerOverflow=off  RndMeth=Floor
  Virtual : Outport
  wires:
  Non-Virtual/1 -> Bus Selector/1
  Bus Creator/1 -> Virtual/1
  Bus Selector/1 -> Data Type Conversion/1  "<ch17>"
  Bus Selector/2 -> Data Type Conversion1/1  "<ch18>"
  Bus Selector/3 -> Data Type Conversion2/1  "<cnt>"
  Bus Selector/4 -> Data Type Conversion3/1  "<cmd>"
  Data Type Conversion2/1 -> Bus Creator/3  "Counts"
  Data Type Conversion3/1 -> Bus Creator/4  "Cmds"
  Data Type Conversion1/1 -> Bus Creator/2  "Ch 18"
  Data Type Conversion/1 -> Bus Creator/1  "Ch 17"

== system ground_sim/Flight Management Unit/Vehicle Management System (VMS)/Variant Subsystem/FMU v2 Beta/Virtual to Non-Virtual Mapping1/Virtual to Non-Virtual Mapping1 ==
  Virtual : Inport
  Bus Creator : BusCreator  Inputs=6
  Bus Selector : BusSelector  OutputSignals=New Data,Lost Frame,Failsafe,Ch 17,Ch 18,Channel Data
  Data Type Conversion{,1..4} (5 alike) : DataTypeConversion  OutDataTypeStr=boolean  SaturateOnIntegerOverflow=off  RndMeth=Floor
  Data Type Conversion5 : DataTypeConversion  OutDataTypeStr=int16  SaturateOnIntegerOverflow=off  RndMeth=Floor
  Non-Virtual : Outport  OutDataTypeStr=Bus: InceptorData
  wires:
  Virtual/1 -> Bus Selector/1
  Bus Creator/1 -> Non-Virtual/1
  Bus Selector/1 -> Data Type Conversion/1  "<New Data>"
  Bus Selector/2 -> Data Type Conversion1/1  "<Lost Frame>"
  Bus Selector/3 -> Data Type Conversion2/1  "<Failsafe>"
  Bus Selector/4 -> Data Type Conversion3/1  "<Ch 17>"
  Bus Selector/5 -> Data Type Conversion4/1  "<Ch 18>"
  Bus Selector/6 -> Data Type Conversion5/1  "<Channel Data>"
  Data Type Conversion/1 -> Bus Creator/1  "new_data"
  Data Type Conversion1/1 -> Bus Creator/2  "lost_frame"
  Data Type Conversion2/1 -> Bus Creator/3  "failsafe"
  Data Type Conversion3/1 -> Bus Creator/4  "ch17"
  Data Type Conversion4/1 -> Bus Creator/5  "ch18"
  Data Type Conversion5/1 -> Bus Creator/6  "ch"

== system ground_sim/Flight Management Unit/Vehicle Management System (VMS)/Variant Subsystem/FMU v2 Beta/Virtual to Non-Virtual Mapping1/Virtual to Non-Virtual Mapping2 ==
  Virtual : Inport
  Bus Creator : BusCreator  Inputs=8
  Bus Selector : BusSelector  OutputSignals=New IMU Data,New Magnetometer Data,IMU Healthy,Magnetometer Healthy,Die Temperature [C],Accelerometer [m/s/s],Gyro [rad/s],Magnetometer [uT]
  Data Type Conversion{,1..3} (4 alike) : DataTypeConversion  OutDataTypeStr=boolean  SaturateOnIntegerOverflow=off  RndMeth=Floor
  Data Type Conversion{4..7} (4 alike) : DataTypeConversion  OutDataTypeStr=single  SaturateOnIntegerOverflow=off  RndMeth=Floor
  Non-Virtual : Outport  OutDataTypeStr=Bus: ImuData
  wires:
  Bus Creator/1 -> Non-Virtual/1
  Virtual/1 -> Bus Selector/1
  Bus Selector/1 -> Data Type Conversion/1  "<New IMU Data>"
  Data Type Conversion/1 -> Bus Creator/1  "new_imu_data"
  Bus Selector/2 -> Data Type Conversion1/1  "<New Magnetometer Data>"
  Data Type Conversion1/1 -> Bus Creator/2  "new_mag_data"
  Bus Selector/3 -> Data Type Conversion2/1  "<IMU Healthy>"
  Data Type Conversion2/1 -> Bus Creator/3  "imu_healthy"
  Bus Selector/4 -> Data Type Conversion3/1  "<Magnetometer Healthy>"
  Data Type Conversion3/1 -> Bus Creator/4  "mag_healthy"
  Bus Selector/5 -> Data Type Conversion4/1  "<Die Temperature [C]>"
  Data Type Conversion4/1 -> Bus Creator/5  "die_temp_c"
  Bus Selector/6 -> Data Type Conversion5/1  "<Accelerometer [m/s/s]>"
  Bus Selector/7 -> Data Type Conversion6/1  "<Gyro [rad/s]>"
  Bus Selector/8 -> Data Type Conversion7/1  "<Magnetometer [uT]>"
  Data Type Conversion5/1 -> Bus Creator/6  "accel_mps2"
  Data Type Conversion6/1 -> Bus Creator/7  "gyro_radps"
  Data Type Conversion7/1 -> Bus Creator/8  "mag_ut"

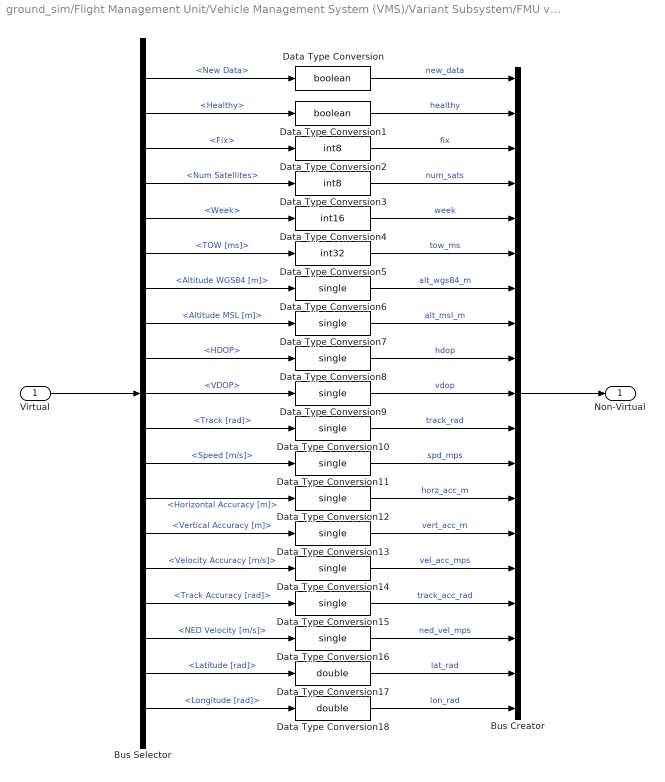
== system ground_sim/Flight Management Unit/Vehicle Management System (VMS)/Variant Subsystem/FMU v2 Beta/Virtual to Non-Virtual Mapping1/Virtual to Non-Virtual Mapping3 ==
  Virtual : Inport
  Bus Creator : BusCreator  Inputs=19
  Bus Selector : BusSelector  OutputSignals=New Data,Healthy,Fix,Num Satellites,Week,TOW [ms],Altitude WGS84 [m],Altitude MSL [m],HDOP,VDOP,Track [rad],Speed [m/s],Horizontal Accuracy [m],Vertical Accuracy [m],Velocity Accuracy [m/s],Track Accuracy [rad],NED Velocity [m/s],Latitude [rad],Longitude [rad]
  Data Type Conversion : DataTypeConversion  OutDataTypeStr=boolean  SaturateOnIntegerOverflow=off  RndMeth=Floor
  Data Type Conversion1 : DataTypeConversion  OutDataTypeStr=boolean  SaturateOnIntegerOverflow=off  RndMeth=Floor
  Data Type Conversion{6..16} (11 alike) : DataTypeConversion  OutDataTypeStr=single  SaturateOnIntegerOverflow=off  RndMeth=Floor
  Data Type Conversion17 : DataTypeConversion  OutDataTypeStr=double  SaturateOnIntegerOverflow=off  RndMeth=Floor
  Data Type Conversion18 : DataTypeConversion  OutDataTypeStr=double  SaturateOnIntegerOverflow=off  RndMeth=Floor
  Data Type Conversion2 : DataTypeConversion  OutDataTypeStr=int8  SaturateOnIntegerOverflow=off  RndMeth=Floor
  Data Type Conversion3 : DataTypeConversion  OutDataTypeStr=int8  SaturateOnIntegerOverflow=off  RndMeth=Floor
  Data Type Conversion4 : DataTypeConversion  OutDataTypeStr=int16  SaturateOnIntegerOverflow=off  RndMeth=Floor
  Data Type Conversion5 : DataTypeConversion  OutDataTypeStr=int32  SaturateOnIntegerOverflow=off  RndMeth=Floor
  Non-Virtual : Outport  OutDataTypeStr=Bus: GnssData
  wires:
  Virtual/1 -> Bus Selector/1
  Bus Creator/1 -> Non-Virtual/1
  Bus Selector/1 -> Data Type Conversion/1  "<New Data>"
  Data Type Conversion/1 -> Bus Creator/1  "new_data"
  Bus Selector/2 -> Data Type Conversion1/1  "<Healthy>"
  Data Type Conversion1/1 -> Bus Creator/2  "healthy"
  Bus Selector/3 -> Data Type Conversion2/1  "<Fix>"
  Data Type Conversion2/1 -> Bus Creator/3  "fix"
  Bus Selector/4 -> Data Type Conversion3/1  "<Num Satellites>"
  Data Type Conversion3/1 -> Bus Creator/4  "num_sats"
  Bus Selector/5 -> Data Type Conversion4/1  "<Week>"
  Data Type Conversion4/1 -> Bus Creator/5  "week"
  Bus Selector/6 -> Data Type Conversion5/1  "<TOW [ms]>"
  Data Type Conversion5/1 -> Bus Creator/6  "tow_ms"
  Bus Selector/7 -> Data Type Conversion6/1  "<Altitude WGS84 [m]>"
  Bus Selector/8 -> Data Type Conversion7/1  "<Altitude MSL [m]>"
  Data Type Conversion6/1 -> Bus Creator/7  "alt_wgs84_m"
  Data Type Conversion7/1 -> Bus Creator/8  "alt_msl_m"
  Bus Selector/9 -> Data Type Conversion8/1  "<HDOP>"
  Bus Selector/10 -> Data Type Conversion9/1  "<VDOP>"
  Data Type Conversion8/1 -> Bus Creator/9  "hdop"
  Data Type Conversion9/1 -> Bus Creator/10  "vdop"
  Bus Selector/11 -> Data Type Conversion10/1  "<Track [rad]>"
  Bus Selector/12 -> Data Type Conversion11/1  "<Speed [m/s]>"
  Data Type Conversion10/1 -> Bus Creator/11  "track_rad"
  Data Type Conversion11/1 -> Bus Creator/12  "spd_mps"
  Bus Selector/13 -> Data Type Conversion12/1  "<Horizontal Accuracy [m]>"
  Bus Selector/14 -> Data Type Conversion13/1  "<Vertical Accuracy [m]>"
  Bus Selector/15 -> Data Type Conversion14/1  "<Velocity Accuracy [m/s]>"
  Bus Selector/16 -> Data Type Conversion15/1  "<Track Accuracy [rad]>"
  Bus Selector/17 -> Data Type Conversion16/1  "<NED Velocity [m/s]>"
  Bus Selector/18 -> Data Type Conversion17/1  "<Latitude [rad]>"
  Bus Selector/19 -> Data Type Conversion18/1  "<Longitude [rad]>"
  Data Type Conversion18/1 -> Bus Creator/19  "lon_rad"
  Data Type Conversion17/1 -> Bus Creator/18  "lat_rad"
  Data Type Conversion16/1 -> Bus Creator/17  "ned_vel_mps"
  Data Type Conversion15/1 -> Bus Creator/16  "track_acc_rad"
  Data Type Conversion14/1 -> Bus Creator/15  "vel_acc_mps"
  Data Type Conversion13/1 -> Bus Creator/14  "vert_acc_m"
  Data Type Conversion12/1 -> Bus Creator/13  "horz_acc_m"

== system ground_sim/Flight Management Unit/Vehicle Management System (VMS)/Variant Subsystem/FMU v2 Beta/Virtual to Non-Virtual Mapping1/Virtual to Non-Virtual Mapping4 ==
  Virtual : Inport
  Bus Creator : BusCreator  Inputs=4
  Bus Selector : BusSelector  OutputSignals=New Data,Healthy,Pressure [Pa],Die Temperature [C]
  Data Type Conversion : DataTypeConversion  OutDataTypeStr=boolean  SaturateOnIntegerOverflow=off  RndMeth=Floor
  Data Type Conversion1 : DataTypeConversion  OutDataTypeStr=boolean  SaturateOnIntegerOverflow=off  RndMeth=Floor
  Data Type Conversion2 : DataTypeConversion  OutDataTypeStr=single  SaturateOnIntegerOverflow=off  RndMeth=Floor
  Data Type Conversion3 : DataTypeConversion  OutDataTypeStr=single  SaturateOnIntegerOverflow=off  RndMeth=Floor
  Non-Virtual : Outport  OutDataTypeStr=Bus: PresData
  wires:
  Bus Creator/1 -> Non-Virtual/1
  Virtual/1 -> Bus Selector/1
  Bus Selector/1 -> Data Type Conversion/1  "<New Data>"
  Data Type Conversion/1 -> Bus Creator/1  "new_data"
  Bus Selector/2 -> Data Type Conversion1/1  "<Healthy>"
  Data Type Conversion1/1 -> Bus Creator/2  "healthy"
  Bus Selector/3 -> Data Type Conversion2/1  "<Pressure [Pa]>"
  Data Type Conversion2/1 -> Bus Creator/3  "pres_pa"
  Bus Selector/4 -> Data Type Conversion3/1  "<Die Temperature [C]>"
  Data Type Conversion3/1 -> Bus Creator/4  "die_temp_c"

== system ground_sim/Flight Management Unit/Vehicle Management System (VMS)/Variant Subsystem/FMU v2 Beta/Virtual to Non-Virtual Mapping1/Virtual to Non-Virtual Mapping5 ==
  Virtual : Inport
  Bus Creator : BusCreator  Inputs=4
  Bus Selector : BusSelector  OutputSignals=New Data,Healthy,Pressure [Pa],Die Temperature [C]
  Data Type Conversion : DataTypeConversion  OutDataTypeStr=boolean  SaturateOnIntegerOverflow=off  RndMeth=Floor
  Data Type Conversion1 : DataTypeConversion  OutDataTypeStr=boolean  SaturateOnIntegerOverflow=off  RndMeth=Floor
  Data Type Conversion2 : DataTypeConversion  OutDataTypeStr=single  SaturateOnIntegerOverflow=off  RndMeth=Floor
  Data Type Conversion3 : DataTypeConversion  OutDataTypeStr=single  SaturateOnIntegerOverflow=off  RndMeth=Floor
  Non-Virtual : Outport  OutDataTypeStr=Bus: PresData
  wires:
  Data Type Conversion3/1 -> Bus Creator/4  "die_temp_c"
  Bus Selector/4 -> Data Type Conversion3/1  "<Die Temperature [C]>"
  Data Type Conversion2/1 -> Bus Creator/3  "pres_pa"
  Bus Selector/3 -> Data Type Conversion2/1  "<Pressure [Pa]>"
  Data Type Conversion1/1 -> Bus Creator/2  "healthy"
  Bus Selector/2 -> Data Type Conversion1/1  "<Healthy>"
  Data Type Conversion/1 -> Bus Creator/1  "new_data"
  Bus Selector/1 -> Data Type Conversion/1  "<New Data>"
  Virtual/1 -> Bus Selector/1
  Bus Creator/1 -> Non-Virtual/1

== system ground_sim/Flight Management Unit/Vehicle Management System (VMS)/Variant Subsystem/FMU v2 Beta/Virtual to Non-Virtual Mapping1/Virtual to Non-Virtual Mapping6 ==
  Virtual : Inport
  Bus Creator : BusCreator  Inputs=1
  Bus Selector : BusSelector  OutputSignals=Voltages
  Data Type Conversion2 : DataTypeConversion  OutDataTypeStr=single  SaturateOnIntegerOverflow=off  RndMeth=Floor
  Non-Virtual : Outport  OutDataTypeStr=Bus: AdcData
  wires:
  Bus Creator/1 -> Non-Virtual/1
  Virtual/1 -> Bus Selector/1
  Data Type Conversion2/1 -> Bus Creator/1  "volt"
  Bus Selector/1 -> Data Type Conversion2/1  "<Voltages>"
